simulink model "PID_controller"  (R2018b)
settings: Solver=VariableStepAuto  StartTime=0.0  StopTime=200  MaxStep=0.01  RelTol=1e-4  EnableMultiTasking=on
values from neighbouring files (symbols this model uses):
  delay = i-1    [main.m]
  period = i*2    [main.m]
libraries: simulink x1
settings Model: Creator=jyotirmoy  LastModifiedBy=saramohamadi
settings DataIOCC: LimitDataPoints=on  SaveOutput=off  SaveTime=off
settings OptimizationCC: ExpressionDepthLimit=2147483647  LifeSpan=1
settings DebuggingCC: UnderspecifiedInitializationDetection=Classic  MergeDetectMultiDrivingBlocksExec=none  FcnCallInpInsideContextMsg=warning  AllowSymbolicDim=off  StateNameClashWarn=warning  SFUnexpectedBacktrackingDiag=warning  SFNoUnconditionalDefaultTransitionDiag=warning  SFExecutionAtInitializationDiag=none
settings SFSimCC: SimUseLocalCustomCode=off
settings RTWCC: RTWUseLocalCustomCode=off
settings CodeAppCC: StateflowObjectComments=on
settings GRTTargetCC: TargetLangStandard=C89/C90 (ANSI)  GeneratePreprocessorConditionals=Disable all  CombineOutputUpdateFcns=off  GRTInterface=on

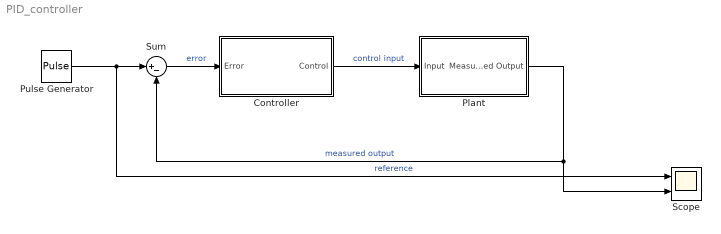
== system PID_controller ==
  Controller : Subsystem
  Plant : Subsystem
  Pulse Generator : DiscretePulseGenerator  PulseType=Time based  Period=period  PulseWidth=50  PhaseDelay=delay
  Scope : Scope  NumInputPorts=2
  Sum : Sum  Inputs=|+-
  wires:
  Pulse Generator/1 -> Scope/1, Sum/1  "reference"
  Plant/1(Measured Output) -> Scope/2, Sum/2  "measured output"
  Sum/1 -> Controller/1(Error)  "error"
  Controller/1(Control) -> Plant/1(Input)  "control input"

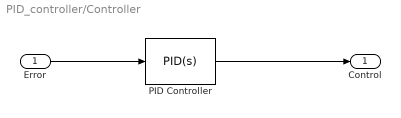
== system PID_controller/Controller ==
  Error : Inport
  PID Controller : simulink/Continuous/PID Controller  Controller=PID  Form=Parallel  TimeDomain=Continuous-time  SampleTime=-1  IntegratorMethod=Forward Euler  FilterMethod=Forward Euler  ControllerParametersSource=internal  P=10  I=1  D=1  UseFilter=on  N=20  TunerSelectOption=Transfer Function Based (PID Tuner App)  InitialConditionSource=internal  InitialConditionForIntegrator=0  InitialConditionForFilter=0  DifferentiatorICPrevScaledInput=0  ExternalReset=none  TrackingMode=off  Kt=1  LimitOutput=off  UpperSaturationLimit=inf  LowerSaturationLimit=-inf  LinearizeAsGain=on  AntiWindupMode=none  Kb=1  POutMin=[]  POutMax=[]  IOutMin=[]  IOutMax=[]  DOutMin=[]  DOutMax=[]  NOutMin=[]  NOutMax=[]  SumOutMin=[]  SumOutMax=[]  SaturationOutMin=[]  SaturationOutMax=[]  PParamMin=[]  PParamMax=[]  IParamMin=[]  IParamMax=[]  DParamMin=[]  DParamMax=[]  NParamMin=[]  NParamMax=[]  KbParamMin=[]  KbParamMax=[]  KtParamMin=[]  KtParamMax=[]  KbOutMin=[]  KbOutMax=[]  KtOutMin=[]  KtOutMax=[]  IntegratorOutMin=[]  IntegratorOutMax=[]  FilterOutMin=[]  FilterOutMax=[]  SumI1OutMin=[]  SumI1OutMax=[]  SumI2OutMin=[]  SumI2OutMax=[]  SumI3OutMin=[]  SumI3OutMax=[]  SumI4OutMin=[]  SumI4OutMax=[]  SumDOutMin=[]  SumDOutMax=[]  DifferentiatorOutMin=[]  DifferentiatorOutMax=[]  FilterDiffOutCoefMin=[]  FilterDiffOutCoefMax=[]  ReciprocalOutMin=[]  ReciprocalOutMax=[]  SumDenOutMin=[]  SumDenOutMax=[]  SumNumOutMin=[]  SumNumOutMax=[]  DivideOutMin=[]  DivideOutMax=[]  IntegratorContinuousStateAttributes=''  IntegratorStateMustResolveToSignalObject=off  IntegratorRTWStateStorageClass=Auto  FilterContinuousStateAttributes=''  FilterStateMustResolveToSignalObject=off  FilterRTWStateStorageClass=Auto  ParallelPVariant=InternalParameters  IdealPVariant=Disabled  IVariant=InternalParameters  DVariant=InternalParameters  IntegratorVariant=Continuous  SatVariant=Disabled  AWVariant=Passthrough  PCopyVariant=Disabled  TRVariant=Disabled  FdbkBlocksVariant=Forward  IdealPFdbkVariant=Disabled  SatFdbkVariant=Disabled  DerivativeFilterVariant=ContFilter  NVariant=InternalParameters  NCopyVariant=Disabled  FilterICVariant=InternalICsFilter  IntegratorICVariant=InternalICs  ExternalResetVariant=Disabled  TRSumVariant=Passthrough  SumFdbkVariant=Disabled  SumVariant=Sum_PID
  Control : Outport
  wires:
  Error/1 -> PID Controller/1
  PID Controller/1 -> Control/1

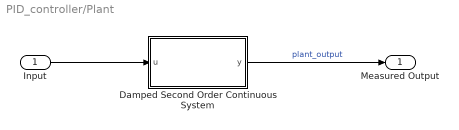
== system PID_controller/Plant ==
  Input : Inport
  Damped Second Order Continuous System : Subsystem  mask{wn=1, zeta=0}
      mask prompts: wn "Undamped natural frequency (wn, rad/s)"; zeta "Damping factor (zeta)"
  Measured Output : Outport
  wires:
  Input/1 -> Damped Second Order Continuous System/1(u)
  Damped Second Order Continuous System/1(y) -> Measured Output/1  "plant_output"

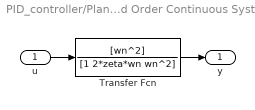
== system PID_controller/Plant/Damped Second Order Continuous System ==
  u : Inport
  Transfer Fcn : TransferFcn  Numerator=[wn^2]  Denominator=[1 2*zeta*wn wn^2]
  y : Outport
  wires:
  Transfer Fcn/1 -> y/1
  u/1 -> Transfer Fcn/1
